simulink model "V2G_FDCC"  (R2024a)
settings: Solver=FixedStepAuto  StartTime=0.0  StopTime=10  FixedStep=1e-5  MaxStep=1.0E-5  RelTol=1e-3
values from neighbouring files (symbols this model uses):
  Batt_Ah = 2000    [main_v2gg2v.m]
  Batt_RespTime = 1    [main_v2gg2v.m]
  Batt_Vnom = 800    [main_v2gg2v.m]
  C_inv = (r*(Pinv/3)*al*(-be+al-1))/(100*Vac_l_rms*Vin_inv*wn*(al-be))    [main_v2gg2v.m]    (also in script.m = 0.00198943678865)
  C_mppt = 20*(Iout_mppt*D_mppt)/(deltaV*fs_mppt)    (= 0.0948148148148)    [main_v2gg2v.m]    (also in script.m)
  C_Vdc = 100*18e-3    (= 1.8)    [main_v2gg2v.m]
  cap_bat = 2000    [main_v2gg2v.m]    (also in script.m)
  Cbat_buck = deltaI_bat/(8*fs_bat*deltaV_bat)    (= 0.00133333333333)    [main_v2gg2v.m]    (also in script.m)
  Cdc = 30e-3    (= 0.03)    [main_v2gg2v.m]    (also in script.m)
  Cdc_boost = 50*Cbat_buck    (= 0.0666666666667)    [main_v2gg2v.m]    (also in script.m)
  Cf = 10*165e-6    (= 0.00165)    [main_v2gg2v.m]
  D = 2    [main_v2gg2v.m]
  Dinv = 0    [main_v2gg2v.m]
  f_grid = 50    [main_v2gg2v.m]
  fg = 50    [main_v2gg2v.m]    (also in script.m)
  H1 = 7    [main_v2gg2v.m]
  H2 = 8    [main_v2gg2v.m]
  H3 = 12    [main_v2gg2v.m]
  Hinv = 0    [main_v2gg2v.m]
  Ki_CC = 1    [main_v2gg2v.m]
  Ki_inner = 5000    [main_v2gg2v.m]
  Ki_outer = 10000    [main_v2gg2v.m]
  Ki_PLL = 10000    [main_v2gg2v.m]
  Kp_CC = 10    [main_v2gg2v.m]
  Kp_inner = 100    [main_v2gg2v.m]
  Kp_outer = 250    [main_v2gg2v.m]
  Kp_PLL = 100    [main_v2gg2v.m]
  L_bat = (Vbat*(Vdc_link-Vbat))/(deltaI_bat*fs_bat*Vdc_link)    (= 0.001875)    [main_v2gg2v.m]    (also in script.m)
  L_mppt = 1*(Vpv*D_mppt)/(deltaI*fs_mppt)    (= 0.000161333333333)    [main_v2gg2v.m]    (also in script.m)
  Lgrid = 1/10*0.69e-3    (= 6.9e-05)    [main_v2gg2v.m]
  Linv = 1/10*0.48e-3    (= 4.8e-05)    [main_v2gg2v.m]
  Lmin_inv = (100*Vac_l_rms*Vin_inv*(al-be))/(wn*r*(Pinv/3)*(-be+al-1))    [main_v2gg2v.m]    (also in script.m = 0.000611154981473)
  LowSat_CC = 0    [main_v2gg2v.m]
  omega = 2*pi*f_grid    (= 314.159265359)    [main_v2gg2v.m]
  Pinv = 2e6    (= 2000000)    [main_v2gg2v.m]    (also in script.m)
  Rd = 1.31    [main_v2gg2v.m]
  Sbase = 1e6    (= 1000000)    [main_v2gg2v.m]    (also in script.m)
  Snom_trafo = 1050e6    (= 1050000000)    [main_v2gg2v.m]
  t_fault_end = t_fault_start + FCT    (= 1.1)    [main_v2gg2v.m]
  t_fault_start = 1    [main_v2gg2v.m]
  Ts = 1e-5    (= 1e-05)    [main_v2gg2v.m]
  UpSat_CC = 1    [main_v2gg2v.m]
  Vac_inv = 800    [main_v2gg2v.m]    (also in script.m)
  Vbase = 345e3    (= 345000)    [main_v2gg2v.m]    (also in script.m)
  Vbat = 750    [main_v2gg2v.m]    (also in script.m)
  Vdc_ref = 1.5e3    (= 1500)    [main_v2gg2v.m]
  wg = 2*pi*fg    (= 314.159265359)    [main_v2gg2v.m]    (also in script.m)
undefined symbols (not defined in the file or in its folder): Acid, D1, Delta, h_PEV, Ibatfault_ref, ibatref, Ion, L12, L13, L23, Lbat, Lbuckboost, Lead, Lithium, R_Vdc, Rbuckboost, Vfault_thresh, vthref
libraries: spsSeriesRLCBranchLib x74, slpidlib x62, spsMosfetLib x50, spsGroundLib x48, spsBatteryLib x31, eeGeneralControl x31, spsPWMGeneratorDCDCLib x29, spsCurrentMeasurementLib x28, spsThreePhaseSeriesRLCBranchLib x21, spsThreePhaseVIMeasurementLib x18, spsIGBTDiodeLib x18, spsVoltageMeasurementLib x14
(part 9 of 11)

== system V2G_FDCC/V2G-G2V-1/5 Charging Stations/Charging Station5 ==
  Ibat_ref : Inport
  Battery : spsBatteryLib/Battery  BatType=Lithium-Ion  ShowTempParam=off  ThermalPreset=no  ShowAgeParam=off  NomV=Batt_Vnom  NomQ=Batt_Ah  SOC=Batt_InitSOC  Batt_Tr=Batt_RespTime  PresetModel=on  MaxQ=2000  MinV=600  FullV=931.1897  Dis_rate=869.5652  R=0.004  Normal_OP=1808.6957  expZone="[864.3087      98.26087]"  current=[6.5 13 32.5]  Units=Time  Tci=20  NomT=20  T2=-30  MaxQ2=4.8  FullV2=7.1  Normal_OP2=5.655  expZone2="[6.58           1]"  Rca=0.6  ti=2000  Dp=0  Neq0=0  Tsim=1e6  Ta1=25  Qeol=5.4*0.9  Reol=0.013333*1.2  Char_age=[2.3478, 3]  Dis_age=[2.3478, 10]  N1=1500  N2=10500  N3=1000  N4=1400  Ta2=45  N5=950
      settings: LibrarySourceBlock=electricdrivelib/Extra Sources/Battery
  Bus Selector : BusSelector  OutputSignals=SOC (%),Current (A),Voltage (V)
  Logical Operator : Logic  Operator=NOT  AllPortsSameDT=off  OutDataTypeStr=boolean
  Mosfet : spsMosfetLib/Mosfet  Ron=0.1  Lon=0  Rd=0.01  Vfd=0  IC=0  Rs=1e5  Cs=inf  Measurements=off
  Mosfet1 : spsMosfetLib/Mosfet  Ron=0.1  Lon=0  Rd=0.01  Vfd=0  IC=0  Rs=1e5  Cs=inf  Measurements=off
  PID Controller4 : slpidlib/PID Controller  Controller=PI  Form=Parallel  TimeDomain=Continuous-time  UseExternalTs=off  SampleTime=-1  IntegratorMethod=Forward Euler  FilterMethod=Forward Euler  ControllerParametersSource=internal  P=Kp_CC  I=Ki_CC  UseKiTs=off  D=0  UseExternalDerivativeSource=off  N=100  UseFilter=on  TunerSelectOption=Transfer Function Based (PID Tuner App)  ZeroCross=off  InitialConditionSource=internal  InitialConditionForIntegrator=0  InitialConditionForFilter=0  DifferentiatorICPrevScaledInput=0  ExternalReset=none  TrackingMode=off  Kt=1  LimitOutput=on  SatLimitsSource=internal  UpperSaturationLimit=UpSat_CC  LowerSaturationLimit=LowSat_CC  LinearizeAsGain=on  AntiWindupMode=none  Kb=1  LimitIntegrator=off  UpperIntegratorSaturationLimit=inf  LowerIntegratorSaturationLimit=-inf  POutMin=[]  POutMax=[]  IOutMin=[]  IOutMax=[]  DOutMin=[]  DOutMax=[]  NOutMin=[]  NOutMax=[]  SumOutMin=[]  SumOutMax=[]  SaturationOutMin=[]  SaturationOutMax=[]  PParamMin=[]  PParamMax=[]  IParamMin=[]  IParamMax=[]  DParamMin=[]  DParamMax=[]  NParamMin=[]  NParamMax=[]  KbParamMin=[]  KbParamMax=[]  KtParamMin=[]  KtParamMax=[]  KbOutMin=[]  KbOutMax=[]  KtOutMin=[]  KtOutMax=[]  IntegratorOutMin=[]  IntegratorOutMax=[]  FilterOutMin=[]  FilterOutMax=[]  SumI1OutMin=[]  SumI1OutMax=[]  SumI2OutMin=[]  SumI2OutMax=[]  SumI3OutMin=[]  SumI3OutMax=[]  SumI4OutMin=[]  SumI4OutMax=[]  SumDOutMin=[]  SumDOutMax=[]  DifferentiatorOutMin=[]  DifferentiatorOutMax=[]  FilterDiffOutCoefMin=[]  FilterDiffOutCoefMax=[]  ReciprocalOutMin=[]  ReciprocalOutMax=[]  SumDenOutMin=[]  SumDenOutMax=[]  SumNumOutMin=[]  SumNumOutMax=[]  DivideOutMin=[]  DivideOutMax=[]  UdiffTsProdOutMin=[]  UdiffTsProdOutMax=[]  NTsProdOutMin=[]  NTsProdOutMax=[]  UintegralTsProdOutMin=[]  UintegralTsProdOutMax=[]  UngainTsProdOutMin=[]  UngainTsProdOutMax=[]  ClampingZeroOutDataTypeStr=Inherit: Inherit via back propagation  ClampingZeroOutMin=[]  ClampingZeroOutMax=[]  FilterDenConstantOutDataTypeStr=Inherit: Inherit via back propagation  FilterDenConstantOutMin=[]  FilterDenConstantOutMax=[]  PCopyOutDataTypeStr=Inherit: Inherit via back propagation  PCopyOutMin=[]  PCopyOutMax=[]  NCopyOutDataTypeStr=Inherit: Inherit via back propagation  NCopyOutMin=[]  NCopyOutMax=[]  IntegratorContinuousStateAttributes=''  IntegratorStateMustResolveToSignalObject=off  IntegratorRTWStateStorageClass=Auto  FilterContinuousStateAttributes=''  FilterStateMustResolveToSignalObject=off  FilterRTWStateStorageClass=Auto  ParallelPVariant=InternalParameters  IdealPVariant=Disabled  IVariant=InternalParameters  DVariant=Disabled  IntegratorVariant=Continuous  SatVariant=Enabled  AWVariant=Passthrough  PCopyVariant=Disabled  TRVariant=Disabled  FdbkBlocksVariant=Forward  IdealPFdbkVariant=Disabled  SatFdbkVariant=Disabled  DerivativeFilterVariant=Disabled  NVariant=Disabled  NCopyVariant=Disabled_SignalSpec  FilterICVariant=Disabled  IntegratorICVariant=InternalICs  ExternalResetVariant=Disabled  TRSumVariant=Passthrough  SumFdbkVariant=Disabled  SumVariant=Sum_PI  TsampFilterVariant=InternalTs  TsampNgainVariant=Passthrough  TsampIntegralVariant=Disabled_SignalSpec  ExternalSaturationOutDataTypeStr=Inherit: Same as second input  DerivativeSourceVariant=Disabled
  PWM Generator (DC-DC) : spsPWMGeneratorDCDCLib/PWM Generator (DC-DC)  Fsw=f_SW  Ts=0
  Series RLC Branch9 : spsSeriesRLCBranchLib/Series RLC Branch  LConnTagsString=__new0  RConnTagsString=__new0  BranchType=L  Resistance=Rbuckboost  Inductance=Lbat  SetiL0=off  InitialCurrent=0  Capacitance=1e-6  Setx0=off  InitialVoltage=0  Measurements=None
  Sum8 : Sum  Inputs=|+-
  Terminator{,1..3} (4 alike) : Terminator
  VDC+ : PMIOPort  Side=Left
  VDC- : PMIOPort  Port=2  Side=Left
  wires:
  Bus Selector/3 -> Terminator3/1  "<Voltage (V)>"
  Bus Selector/2 -> Terminator2/1, [Ibat]  "<Current (A)>"
  [Buck] -> Mosfet/1
  Battery/1 -> Terminator/1, Bus Selector/1
  [Boost] -> Mosfet1/1
  Bus Selector/1 -> Terminator1/1  "<SOC (%)>"
  Logical Operator/1 -> [Boost]
  Ibat_ref/1 -> Sum8/2
  PID Controller4/1 -> PWM Generator (DC-DC)/1
  [Ibat] -> Sum8/1
  Sum8/1 -> PID Controller4/1
  PWM Generator (DC-DC)/1 -> Logical Operator/1, [Buck]
  connections:
  VDC-/RConn1 -- Battery/LConn2 -- Mosfet1/RConn1
  Mosfet/LConn1 -- VDC+/RConn1
  Mosfet1/LConn1 -- Series RLC Branch9/RConn1 -- Mosfet/RConn1
  Battery/LConn1 -- Series RLC Branch9/LConn1

== system V2G_FDCC/V2G-G2V-1/5 Charging Stations/Charging Station6 ==
  Ibat_ref : Inport
  Battery : spsBatteryLib/Battery  BatType=Lithium-Ion  ShowTempParam=off  ThermalPreset=no  ShowAgeParam=off  NomV=Batt_Vnom  NomQ=Batt_Ah  SOC=Batt_InitSOC  Batt_Tr=Batt_RespTime  PresetModel=on  MaxQ=2000  MinV=600  FullV=931.1897  Dis_rate=869.5652  R=0.004  Normal_OP=1808.6957  expZone="[864.3087      98.26087]"  current=[6.5 13 32.5]  Units=Time  Tci=20  NomT=20  T2=-30  MaxQ2=4.8  FullV2=7.1  Normal_OP2=5.655  expZone2="[6.58           1]"  Rca=0.6  ti=2000  Dp=0  Neq0=0  Tsim=1e6  Ta1=25  Qeol=5.4*0.9  Reol=0.013333*1.2  Char_age=[2.3478, 3]  Dis_age=[2.3478, 10]  N1=1500  N2=10500  N3=1000  N4=1400  Ta2=45  N5=950
      settings: LibrarySourceBlock=electricdrivelib/Extra Sources/Battery
  Bus Selector : BusSelector  OutputSignals=SOC (%),Current (A),Voltage (V)
  Logical Operator : Logic  Operator=NOT  AllPortsSameDT=off  OutDataTypeStr=boolean
  Mosfet : spsMosfetLib/Mosfet  Ron=0.1  Lon=0  Rd=0.01  Vfd=0  IC=0  Rs=1e5  Cs=inf  Measurements=off
  Mosfet1 : spsMosfetLib/Mosfet  Ron=0.1  Lon=0  Rd=0.01  Vfd=0  IC=0  Rs=1e5  Cs=inf  Measurements=off
  PID Controller4 : slpidlib/PID Controller  Controller=PI  Form=Parallel  TimeDomain=Continuous-time  UseExternalTs=off  SampleTime=-1  IntegratorMethod=Forward Euler  FilterMethod=Forward Euler  ControllerParametersSource=internal  P=Kp_CC  I=Ki_CC  UseKiTs=off  D=0  UseExternalDerivativeSource=off  N=100  UseFilter=on  TunerSelectOption=Transfer Function Based (PID Tuner App)  ZeroCross=off  InitialConditionSource=internal  InitialConditionForIntegrator=0  InitialConditionForFilter=0  DifferentiatorICPrevScaledInput=0  ExternalReset=none  TrackingMode=off  Kt=1  LimitOutput=on  SatLimitsSource=internal  UpperSaturationLimit=UpSat_CC  LowerSaturationLimit=LowSat_CC  LinearizeAsGain=on  AntiWindupMode=none  Kb=1  LimitIntegrator=off  UpperIntegratorSaturationLimit=inf  LowerIntegratorSaturationLimit=-inf  POutMin=[]  POutMax=[]  IOutMin=[]  IOutMax=[]  DOutMin=[]  DOutMax=[]  NOutMin=[]  NOutMax=[]  SumOutMin=[]  SumOutMax=[]  SaturationOutMin=[]  SaturationOutMax=[]  PParamMin=[]  PParamMax=[]  IParamMin=[]  IParamMax=[]  DParamMin=[]  DParamMax=[]  NParamMin=[]  NParamMax=[]  KbParamMin=[]  KbParamMax=[]  KtParamMin=[]  KtParamMax=[]  KbOutMin=[]  KbOutMax=[]  KtOutMin=[]  KtOutMax=[]  IntegratorOutMin=[]  IntegratorOutMax=[]  FilterOutMin=[]  FilterOutMax=[]  SumI1OutMin=[]  SumI1OutMax=[]  SumI2OutMin=[]  SumI2OutMax=[]  SumI3OutMin=[]  SumI3OutMax=[]  SumI4OutMin=[]  SumI4OutMax=[]  SumDOutMin=[]  SumDOutMax=[]  DifferentiatorOutMin=[]  DifferentiatorOutMax=[]  FilterDiffOutCoefMin=[]  FilterDiffOutCoefMax=[]  ReciprocalOutMin=[]  ReciprocalOutMax=[]  SumDenOutMin=[]  SumDenOutMax=[]  SumNumOutMin=[]  SumNumOutMax=[]  DivideOutMin=[]  DivideOutMax=[]  UdiffTsProdOutMin=[]  UdiffTsProdOutMax=[]  NTsProdOutMin=[]  NTsProdOutMax=[]  UintegralTsProdOutMin=[]  UintegralTsProdOutMax=[]  UngainTsProdOutMin=[]  UngainTsProdOutMax=[]  ClampingZeroOutDataTypeStr=Inherit: Inherit via back propagation  ClampingZeroOutMin=[]  ClampingZeroOutMax=[]  FilterDenConstantOutDataTypeStr=Inherit: Inherit via back propagation  FilterDenConstantOutMin=[]  FilterDenConstantOutMax=[]  PCopyOutDataTypeStr=Inherit: Inherit via back propagation  PCopyOutMin=[]  PCopyOutMax=[]  NCopyOutDataTypeStr=Inherit: Inherit via back propagation  NCopyOutMin=[]  NCopyOutMax=[]  IntegratorContinuousStateAttributes=''  IntegratorStateMustResolveToSignalObject=off  IntegratorRTWStateStorageClass=Auto  FilterContinuousStateAttributes=''  FilterStateMustResolveToSignalObject=off  FilterRTWStateStorageClass=Auto  ParallelPVariant=InternalParameters  IdealPVariant=Disabled  IVariant=InternalParameters  DVariant=Disabled  IntegratorVariant=Continuous  SatVariant=Enabled  AWVariant=Passthrough  PCopyVariant=Disabled  TRVariant=Disabled  FdbkBlocksVariant=Forward  IdealPFdbkVariant=Disabled  SatFdbkVariant=Disabled  DerivativeFilterVariant=Disabled  NVariant=Disabled  NCopyVariant=Disabled_SignalSpec  FilterICVariant=Disabled  IntegratorICVariant=InternalICs  ExternalResetVariant=Disabled  TRSumVariant=Passthrough  SumFdbkVariant=Disabled  SumVariant=Sum_PI  TsampFilterVariant=InternalTs  TsampNgainVariant=Passthrough  TsampIntegralVariant=Disabled_SignalSpec  ExternalSaturationOutDataTypeStr=Inherit: Same as second input  DerivativeSourceVariant=Disabled
  PWM Generator (DC-DC) : spsPWMGeneratorDCDCLib/PWM Generator (DC-DC)  Fsw=f_SW  Ts=0
  Series RLC Branch9 : spsSeriesRLCBranchLib/Series RLC Branch  LConnTagsString=__new0  RConnTagsString=__new0  BranchType=L  Resistance=Rbuckboost  Inductance=Lbat  SetiL0=off  InitialCurrent=0  Capacitance=1e-6  Setx0=off  InitialVoltage=0  Measurements=None
  Sum8 : Sum  Inputs=|+-
  Terminator{,1..3} (4 alike) : Terminator
  VDC+ : PMIOPort  Side=Left
  VDC- : PMIOPort  Port=2  Side=Left
  wires:
  Bus Selector/3 -> Terminator3/1  "<Voltage (V)>"
  Bus Selector/2 -> Terminator2/1, [Ibat]  "<Current (A)>"
  [Buck] -> Mosfet/1
  Battery/1 -> Terminator/1, Bus Selector/1
  [Boost] -> Mosfet1/1
  Bus Selector/1 -> Terminator1/1  "<SOC (%)>"
  Logical Operator/1 -> [Boost]
  Ibat_ref/1 -> Sum8/2
  PID Controller4/1 -> PWM Generator (DC-DC)/1
  [Ibat] -> Sum8/1
  Sum8/1 -> PID Controller4/1
  PWM Generator (DC-DC)/1 -> Logical Operator/1, [Buck]
  connections:
  VDC-/RConn1 -- Battery/LConn2 -- Mosfet1/RConn1
  Mosfet/LConn1 -- VDC+/RConn1
  Mosfet1/LConn1 -- Series RLC Branch9/RConn1 -- Mosfet/RConn1
  Battery/LConn1 -- Series RLC Branch9/LConn1

== system V2G_FDCC/V2G-G2V-1/5 Charging Stations/Charging Station7 ==
  Ibat_ref : Inport
  Battery : spsBatteryLib/Battery  BatType=Lithium-Ion  ShowTempParam=off  ThermalPreset=no  ShowAgeParam=off  NomV=Batt_Vnom  NomQ=Batt_Ah  SOC=Batt_InitSOC  Batt_Tr=Batt_RespTime  PresetModel=on  MaxQ=2000  MinV=600  FullV=931.1897  Dis_rate=869.5652  R=0.004  Normal_OP=1808.6957  expZone="[864.3087      98.26087]"  current=[6.5 13 32.5]  Units=Time  Tci=20  NomT=20  T2=-30  MaxQ2=4.8  FullV2=7.1  Normal_OP2=5.655  expZone2="[6.58           1]"  Rca=0.6  ti=2000  Dp=0  Neq0=0  Tsim=1e6  Ta1=25  Qeol=5.4*0.9  Reol=0.013333*1.2  Char_age=[2.3478, 3]  Dis_age=[2.3478, 10]  N1=1500  N2=10500  N3=1000  N4=1400  Ta2=45  N5=950
      settings: LibrarySourceBlock=electricdrivelib/Extra Sources/Battery
  Bus Selector : BusSelector  OutputSignals=SOC (%),Current (A),Voltage (V)
  Logical Operator : Logic  Operator=NOT  AllPortsSameDT=off  OutDataTypeStr=boolean
  Mosfet : spsMosfetLib/Mosfet  Ron=0.1  Lon=0  Rd=0.01  Vfd=0  IC=0  Rs=1e5  Cs=inf  Measurements=off
  Mosfet1 : spsMosfetLib/Mosfet  Ron=0.1  Lon=0  Rd=0.01  Vfd=0  IC=0  Rs=1e5  Cs=inf  Measurements=off
  PID Controller4 : slpidlib/PID Controller  Controller=PI  Form=Parallel  TimeDomain=Continuous-time  UseExternalTs=off  SampleTime=-1  IntegratorMethod=Forward Euler  FilterMethod=Forward Euler  ControllerParametersSource=internal  P=Kp_CC  I=Ki_CC  UseKiTs=off  D=0  UseExternalDerivativeSource=off  N=100  UseFilter=on  TunerSelectOption=Transfer Function Based (PID Tuner App)  ZeroCross=off  InitialConditionSource=internal  InitialConditionForIntegrator=0  InitialConditionForFilter=0  DifferentiatorICPrevScaledInput=0  ExternalReset=none  TrackingMode=off  Kt=1  LimitOutput=on  SatLimitsSource=internal  UpperSaturationLimit=UpSat_CC  LowerSaturationLimit=LowSat_CC  LinearizeAsGain=on  AntiWindupMode=none  Kb=1  LimitIntegrator=off  UpperIntegratorSaturationLimit=inf  LowerIntegratorSaturationLimit=-inf  POutMin=[]  POutMax=[]  IOutMin=[]  IOutMax=[]  DOutMin=[]  DOutMax=[]  NOutMin=[]  NOutMax=[]  SumOutMin=[]  SumOutMax=[]  SaturationOutMin=[]  SaturationOutMax=[]  PParamMin=[]  PParamMax=[]  IParamMin=[]  IParamMax=[]  DParamMin=[]  DParamMax=[]  NParamMin=[]  NParamMax=[]  KbParamMin=[]  KbParamMax=[]  KtParamMin=[]  KtParamMax=[]  KbOutMin=[]  KbOutMax=[]  KtOutMin=[]  KtOutMax=[]  IntegratorOutMin=[]  IntegratorOutMax=[]  FilterOutMin=[]  FilterOutMax=[]  SumI1OutMin=[]  SumI1OutMax=[]  SumI2OutMin=[]  SumI2OutMax=[]  SumI3OutMin=[]  SumI3OutMax=[]  SumI4OutMin=[]  SumI4OutMax=[]  SumDOutMin=[]  SumDOutMax=[]  DifferentiatorOutMin=[]  DifferentiatorOutMax=[]  FilterDiffOutCoefMin=[]  FilterDiffOutCoefMax=[]  ReciprocalOutMin=[]  ReciprocalOutMax=[]  SumDenOutMin=[]  SumDenOutMax=[]  SumNumOutMin=[]  SumNumOutMax=[]  DivideOutMin=[]  DivideOutMax=[]  UdiffTsProdOutMin=[]  UdiffTsProdOutMax=[]  NTsProdOutMin=[]  NTsProdOutMax=[]  UintegralTsProdOutMin=[]  UintegralTsProdOutMax=[]  UngainTsProdOutMin=[]  UngainTsProdOutMax=[]  ClampingZeroOutDataTypeStr=Inherit: Inherit via back propagation  ClampingZeroOutMin=[]  ClampingZeroOutMax=[]  FilterDenConstantOutDataTypeStr=Inherit: Inherit via back propagation  FilterDenConstantOutMin=[]  FilterDenConstantOutMax=[]  PCopyOutDataTypeStr=Inherit: Inherit via back propagation  PCopyOutMin=[]  PCopyOutMax=[]  NCopyOutDataTypeStr=Inherit: Inherit via back propagation  NCopyOutMin=[]  NCopyOutMax=[]  IntegratorContinuousStateAttributes=''  IntegratorStateMustResolveToSignalObject=off  IntegratorRTWStateStorageClass=Auto  FilterContinuousStateAttributes=''  FilterStateMustResolveToSignalObject=off  FilterRTWStateStorageClass=Auto  ParallelPVariant=InternalParameters  IdealPVariant=Disabled  IVariant=InternalParameters  DVariant=Disabled  IntegratorVariant=Continuous  SatVariant=Enabled  AWVariant=Passthrough  PCopyVariant=Disabled  TRVariant=Disabled  FdbkBlocksVariant=Forward  IdealPFdbkVariant=Disabled  SatFdbkVariant=Disabled  DerivativeFilterVariant=Disabled  NVariant=Disabled  NCopyVariant=Disabled_SignalSpec  FilterICVariant=Disabled  IntegratorICVariant=InternalICs  ExternalResetVariant=Disabled  TRSumVariant=Passthrough  SumFdbkVariant=Disabled  SumVariant=Sum_PI  TsampFilterVariant=InternalTs  TsampNgainVariant=Passthrough  TsampIntegralVariant=Disabled_SignalSpec  ExternalSaturationOutDataTypeStr=Inherit: Same as second input  DerivativeSourceVariant=Disabled
  PWM Generator (DC-DC) : spsPWMGeneratorDCDCLib/PWM Generator (DC-DC)  Fsw=f_SW  Ts=0
  Series RLC Branch9 : spsSeriesRLCBranchLib/Series RLC Branch  LConnTagsString=__new0  RConnTagsString=__new0  BranchType=L  Resistance=Rbuckboost  Inductance=Lbat  SetiL0=off  InitialCurrent=0  Capacitance=1e-6  Setx0=off  InitialVoltage=0  Measurements=None
  Sum8 : Sum  Inputs=|+-
  Terminator{,1..3} (4 alike) : Terminator
  VDC+ : PMIOPort  Side=Left
  VDC- : PMIOPort  Port=2  Side=Left
  wires:
  Bus Selector/3 -> Terminator3/1  "<Voltage (V)>"
  Bus Selector/2 -> Terminator2/1, [Ibat]  "<Current (A)>"
  [Buck] -> Mosfet/1
  Battery/1 -> Terminator/1, Bus Selector/1
  [Boost] -> Mosfet1/1
  Bus Selector/1 -> Terminator1/1  "<SOC (%)>"
  Logical Operator/1 -> [Boost]
  Ibat_ref/1 -> Sum8/2
  PID Controller4/1 -> PWM Generator (DC-DC)/1
  [Ibat] -> Sum8/1
  Sum8/1 -> PID Controller4/1
  PWM Generator (DC-DC)/1 -> Logical Operator/1, [Buck]
  connections:
  VDC-/RConn1 -- Battery/LConn2 -- Mosfet1/RConn1
  Mosfet/LConn1 -- VDC+/RConn1
  Mosfet1/LConn1 -- Series RLC Branch9/RConn1 -- Mosfet/RConn1
  Battery/LConn1 -- Series RLC Branch9/LConn1

== system V2G_FDCC/V2G-G2V-1/5 Charging Stations/Charging Station8 ==
  Ibat_ref : Inport
  Battery : spsBatteryLib/Battery  BatType=Lithium-Ion  ShowTempParam=off  ThermalPreset=no  ShowAgeParam=off  NomV=Batt_Vnom  NomQ=Batt_Ah  SOC=Batt_InitSOC  Batt_Tr=Batt_RespTime  PresetModel=on  MaxQ=2000  MinV=600  FullV=931.1897  Dis_rate=869.5652  R=0.004  Normal_OP=1808.6957  expZone="[864.3087      98.26087]"  current=[6.5 13 32.5]  Units=Time  Tci=20  NomT=20  T2=-30  MaxQ2=4.8  FullV2=7.1  Normal_OP2=5.655  expZone2="[6.58           1]"  Rca=0.6  ti=2000  Dp=0  Neq0=0  Tsim=1e6  Ta1=25  Qeol=5.4*0.9  Reol=0.013333*1.2  Char_age=[2.3478, 3]  Dis_age=[2.3478, 10]  N1=1500  N2=10500  N3=1000  N4=1400  Ta2=45  N5=950
      settings: LibrarySourceBlock=electricdrivelib/Extra Sources/Battery
  Bus Selector : BusSelector  OutputSignals=SOC (%),Current (A),Voltage (V)
  Logical Operator : Logic  Operator=NOT  AllPortsSameDT=off  OutDataTypeStr=boolean
  Mosfet : spsMosfetLib/Mosfet  Ron=0.1  Lon=0  Rd=0.01  Vfd=0  IC=0  Rs=1e5  Cs=inf  Measurements=off
  Mosfet1 : spsMosfetLib/Mosfet  Ron=0.1  Lon=0  Rd=0.01  Vfd=0  IC=0  Rs=1e5  Cs=inf  Measurements=off
  PID Controller4 : slpidlib/PID Controller  Controller=PI  Form=Parallel  TimeDomain=Continuous-time  UseExternalTs=off  SampleTime=-1  IntegratorMethod=Forward Euler  FilterMethod=Forward Euler  ControllerParametersSource=internal  P=Kp_CC  I=Ki_CC  UseKiTs=off  D=0  UseExternalDerivativeSource=off  N=100  UseFilter=on  TunerSelectOption=Transfer Function Based (PID Tuner App)  ZeroCross=off  InitialConditionSource=internal  InitialConditionForIntegrator=0  InitialConditionForFilter=0  DifferentiatorICPrevScaledInput=0  ExternalReset=none  TrackingMode=off  Kt=1  LimitOutput=on  SatLimitsSource=internal  UpperSaturationLimit=UpSat_CC  LowerSaturationLimit=LowSat_CC  LinearizeAsGain=on  AntiWindupMode=none  Kb=1  LimitIntegrator=off  UpperIntegratorSaturationLimit=inf  LowerIntegratorSaturationLimit=-inf  POutMin=[]  POutMax=[]  IOutMin=[]  IOutMax=[]  DOutMin=[]  DOutMax=[]  NOutMin=[]  NOutMax=[]  SumOutMin=[]  SumOutMax=[]  SaturationOutMin=[]  SaturationOutMax=[]  PParamMin=[]  PParamMax=[]  IParamMin=[]  IParamMax=[]  DParamMin=[]  DParamMax=[]  NParamMin=[]  NParamMax=[]  KbParamMin=[]  KbParamMax=[]  KtParamMin=[]  KtParamMax=[]  KbOutMin=[]  KbOutMax=[]  KtOutMin=[]  KtOutMax=[]  IntegratorOutMin=[]  IntegratorOutMax=[]  FilterOutMin=[]  FilterOutMax=[]  SumI1OutMin=[]  SumI1OutMax=[]  SumI2OutMin=[]  SumI2OutMax=[]  SumI3OutMin=[]  SumI3OutMax=[]  SumI4OutMin=[]  SumI4OutMax=[]  SumDOutMin=[]  SumDOutMax=[]  DifferentiatorOutMin=[]  DifferentiatorOutMax=[]  FilterDiffOutCoefMin=[]  FilterDiffOutCoefMax=[]  ReciprocalOutMin=[]  ReciprocalOutMax=[]  SumDenOutMin=[]  SumDenOutMax=[]  SumNumOutMin=[]  SumNumOutMax=[]  DivideOutMin=[]  DivideOutMax=[]  UdiffTsProdOutMin=[]  UdiffTsProdOutMax=[]  NTsProdOutMin=[]  NTsProdOutMax=[]  UintegralTsProdOutMin=[]  UintegralTsProdOutMax=[]  UngainTsProdOutMin=[]  UngainTsProdOutMax=[]  ClampingZeroOutDataTypeStr=Inherit: Inherit via back propagation  ClampingZeroOutMin=[]  ClampingZeroOutMax=[]  FilterDenConstantOutDataTypeStr=Inherit: Inherit via back propagation  FilterDenConstantOutMin=[]  FilterDenConstantOutMax=[]  PCopyOutDataTypeStr=Inherit: Inherit via back propagation  PCopyOutMin=[]  PCopyOutMax=[]  NCopyOutDataTypeStr=Inherit: Inherit via back propagation  NCopyOutMin=[]  NCopyOutMax=[]  IntegratorContinuousStateAttributes=''  IntegratorStateMustResolveToSignalObject=off  IntegratorRTWStateStorageClass=Auto  FilterContinuousStateAttributes=''  FilterStateMustResolveToSignalObject=off  FilterRTWStateStorageClass=Auto  ParallelPVariant=InternalParameters  IdealPVariant=Disabled  IVariant=InternalParameters  DVariant=Disabled  IntegratorVariant=Continuous  SatVariant=Enabled  AWVariant=Passthrough  PCopyVariant=Disabled  TRVariant=Disabled  FdbkBlocksVariant=Forward  IdealPFdbkVariant=Disabled  SatFdbkVariant=Disabled  DerivativeFilterVariant=Disabled  NVariant=Disabled  NCopyVariant=Disabled_SignalSpec  FilterICVariant=Disabled  IntegratorICVariant=InternalICs  ExternalResetVariant=Disabled  TRSumVariant=Passthrough  SumFdbkVariant=Disabled  SumVariant=Sum_PI  TsampFilterVariant=InternalTs  TsampNgainVariant=Passthrough  TsampIntegralVariant=Disabled_SignalSpec  ExternalSaturationOutDataTypeStr=Inherit: Same as second input  DerivativeSourceVariant=Disabled
  PWM Generator (DC-DC) : spsPWMGeneratorDCDCLib/PWM Generator (DC-DC)  Fsw=f_SW  Ts=0
  Series RLC Branch9 : spsSeriesRLCBranchLib/Series RLC Branch  LConnTagsString=__new0  RConnTagsString=__new0  BranchType=L  Resistance=Rbuckboost  Inductance=Lbat  SetiL0=off  InitialCurrent=0  Capacitance=1e-6  Setx0=off  InitialVoltage=0  Measurements=None
  Sum8 : Sum  Inputs=|+-
  Terminator{,1..3} (4 alike) : Terminator
  VDC+ : PMIOPort  Side=Left
  VDC- : PMIOPort  Port=2  Side=Left
  wires:
  Bus Selector/3 -> Terminator3/1  "<Voltage (V)>"
  Bus Selector/2 -> Terminator2/1, [Ibat]  "<Current (A)>"
  [Buck] -> Mosfet/1
  Battery/1 -> Terminator/1, Bus Selector/1
  [Boost] -> Mosfet1/1
  Bus Selector/1 -> Terminator1/1  "<SOC (%)>"
  Logical Operator/1 -> [Boost]
  Ibat_ref/1 -> Sum8/2
  PID Controller4/1 -> PWM Generator (DC-DC)/1
  [Ibat] -> Sum8/1
  Sum8/1 -> PID Controller4/1
  PWM Generator (DC-DC)/1 -> Logical Operator/1, [Buck]
  connections:
  VDC-/RConn1 -- Battery/LConn2 -- Mosfet1/RConn1
  Mosfet/LConn1 -- VDC+/RConn1
  Mosfet1/LConn1 -- Series RLC Branch9/RConn1 -- Mosfet/RConn1
  Battery/LConn1 -- Series RLC Branch9/LConn1

== system V2G_FDCC/V2G-G2V-1/5 Charging Stations/Charging Station9 ==
  Ibat_ref : Inport
  Battery : spsBatteryLib/Battery  BatType=Lithium-Ion  ShowTempParam=off  ThermalPreset=no  ShowAgeParam=off  NomV=Batt_Vnom  NomQ=Batt_Ah  SOC=Batt_InitSOC  Batt_Tr=Batt_RespTime  PresetModel=on  MaxQ=2000  MinV=600  FullV=931.1897  Dis_rate=869.5652  R=0.004  Normal_OP=1808.6957  expZone="[864.3087      98.26087]"  current=[6.5 13 32.5]  Units=Time  Tci=20  NomT=20  T2=-30  MaxQ2=4.8  FullV2=7.1  Normal_OP2=5.655  expZone2="[6.58           1]"  Rca=0.6  ti=2000  Dp=0  Neq0=0  Tsim=1e6  Ta1=25  Qeol=5.4*0.9  Reol=0.013333*1.2  Char_age=[2.3478, 3]  Dis_age=[2.3478, 10]  N1=1500  N2=10500  N3=1000  N4=1400  Ta2=45  N5=950
      settings: LibrarySourceBlock=electricdrivelib/Extra Sources/Battery
  Bus Selector : BusSelector  OutputSignals=SOC (%),Current (A),Voltage (V)
  Logical Operator : Logic  Operator=NOT  AllPortsSameDT=off  OutDataTypeStr=boolean
  Mosfet : spsMosfetLib/Mosfet  Ron=0.1  Lon=0  Rd=0.01  Vfd=0  IC=0  Rs=1e5  Cs=inf  Measurements=off
  Mosfet1 : spsMosfetLib/Mosfet  Ron=0.1  Lon=0  Rd=0.01  Vfd=0  IC=0  Rs=1e5  Cs=inf  Measurements=off
  PID Controller4 : slpidlib/PID Controller  Controller=PI  Form=Parallel  TimeDomain=Continuous-time  UseExternalTs=off  SampleTime=-1  IntegratorMethod=Forward Euler  FilterMethod=Forward Euler  ControllerParametersSource=internal  P=Kp_CC  I=Ki_CC  UseKiTs=off  D=0  UseExternalDerivativeSource=off  N=100  UseFilter=on  TunerSelectOption=Transfer Function Based (PID Tuner App)  ZeroCross=off  InitialConditionSource=internal  InitialConditionForIntegrator=0  InitialConditionForFilter=0  DifferentiatorICPrevScaledInput=0  ExternalReset=none  TrackingMode=off  Kt=1  LimitOutput=on  SatLimitsSource=internal  UpperSaturationLimit=UpSat_CC  LowerSaturationLimit=LowSat_CC  LinearizeAsGain=on  AntiWindupMode=none  Kb=1  LimitIntegrator=off  UpperIntegratorSaturationLimit=inf  LowerIntegratorSaturationLimit=-inf  POutMin=[]  POutMax=[]  IOutMin=[]  IOutMax=[]  DOutMin=[]  DOutMax=[]  NOutMin=[]  NOutMax=[]  SumOutMin=[]  SumOutMax=[]  SaturationOutMin=[]  SaturationOutMax=[]  PParamMin=[]  PParamMax=[]  IParamMin=[]  IParamMax=[]  DParamMin=[]  DParamMax=[]  NParamMin=[]  NParamMax=[]  KbParamMin=[]  KbParamMax=[]  KtParamMin=[]  KtParamMax=[]  KbOutMin=[]  KbOutMax=[]  KtOutMin=[]  KtOutMax=[]  IntegratorOutMin=[]  IntegratorOutMax=[]  FilterOutMin=[]  FilterOutMax=[]  SumI1OutMin=[]  SumI1OutMax=[]  SumI2OutMin=[]  SumI2OutMax=[]  SumI3OutMin=[]  SumI3OutMax=[]  SumI4OutMin=[]  SumI4OutMax=[]  SumDOutMin=[]  SumDOutMax=[]  DifferentiatorOutMin=[]  DifferentiatorOutMax=[]  FilterDiffOutCoefMin=[]  FilterDiffOutCoefMax=[]  ReciprocalOutMin=[]  ReciprocalOutMax=[]  SumDenOutMin=[]  SumDenOutMax=[]  SumNumOutMin=[]  SumNumOutMax=[]  DivideOutMin=[]  DivideOutMax=[]  UdiffTsProdOutMin=[]  UdiffTsProdOutMax=[]  NTsProdOutMin=[]  NTsProdOutMax=[]  UintegralTsProdOutMin=[]  UintegralTsProdOutMax=[]  UngainTsProdOutMin=[]  UngainTsProdOutMax=[]  ClampingZeroOutDataTypeStr=Inherit: Inherit via back propagation  ClampingZeroOutMin=[]  ClampingZeroOutMax=[]  FilterDenConstantOutDataTypeStr=Inherit: Inherit via back propagation  FilterDenConstantOutMin=[]  FilterDenConstantOutMax=[]  PCopyOutDataTypeStr=Inherit: Inherit via back propagation  PCopyOutMin=[]  PCopyOutMax=[]  NCopyOutDataTypeStr=Inherit: Inherit via back propagation  NCopyOutMin=[]  NCopyOutMax=[]  IntegratorContinuousStateAttributes=''  IntegratorStateMustResolveToSignalObject=off  IntegratorRTWStateStorageClass=Auto  FilterContinuousStateAttributes=''  FilterStateMustResolveToSignalObject=off  FilterRTWStateStorageClass=Auto  ParallelPVariant=InternalParameters  IdealPVariant=Disabled  IVariant=InternalParameters  DVariant=Disabled  IntegratorVariant=Continuous  SatVariant=Enabled  AWVariant=Passthrough  PCopyVariant=Disabled  TRVariant=Disabled  FdbkBlocksVariant=Forward  IdealPFdbkVariant=Disabled  SatFdbkVariant=Disabled  DerivativeFilterVariant=Disabled  NVariant=Disabled  NCopyVariant=Disabled_SignalSpec  FilterICVariant=Disabled  IntegratorICVariant=InternalICs  ExternalResetVariant=Disabled  TRSumVariant=Passthrough  SumFdbkVariant=Disabled  SumVariant=Sum_PI  TsampFilterVariant=InternalTs  TsampNgainVariant=Passthrough  TsampIntegralVariant=Disabled_SignalSpec  ExternalSaturationOutDataTypeStr=Inherit: Same as second input  DerivativeSourceVariant=Disabled
  PWM Generator (DC-DC) : spsPWMGeneratorDCDCLib/PWM Generator (DC-DC)  Fsw=f_SW  Ts=0
  Series RLC Branch9 : spsSeriesRLCBranchLib/Series RLC Branch  LConnTagsString=__new0  RConnTagsString=__new0  BranchType=L  Resistance=Rbuckboost  Inductance=Lbat  SetiL0=off  InitialCurrent=0  Capacitance=1e-6  Setx0=off  InitialVoltage=0  Measurements=None
  Sum8 : Sum  Inputs=|+-
  Terminator{,1..3} (4 alike) : Terminator
  VDC+ : PMIOPort  Side=Left
  VDC- : PMIOPort  Port=2  Side=Left
  wires:
  Bus Selector/3 -> Terminator3/1  "<Voltage (V)>"
  Bus Selector/2 -> Terminator2/1, [Ibat]  "<Current (A)>"
  [Buck] -> Mosfet/1
  Battery/1 -> Terminator/1, Bus Selector/1
  [Boost] -> Mosfet1/1
  Bus Selector/1 -> Terminator1/1  "<SOC (%)>"
  Logical Operator/1 -> [Boost]
  Ibat_ref/1 -> Sum8/2
  PID Controller4/1 -> PWM Generator (DC-DC)/1
  [Ibat] -> Sum8/1
  Sum8/1 -> PID Controller4/1
  PWM Generator (DC-DC)/1 -> Logical Operator/1, [Buck]
  connections:
  VDC-/RConn1 -- Battery/LConn2 -- Mosfet1/RConn1
  Mosfet/LConn1 -- VDC+/RConn1
  Mosfet1/LConn1 -- Series RLC Branch9/RConn1 -- Mosfet/RConn1
  Battery/LConn1 -- Series RLC Branch9/LConn1

== system V2G_FDCC/V2G-G2V-1/AC//DC Converter/Subsystem ==
  PWM1 : Inport
  PWM2 : Inport  Port=2
  PWM3 : Inport  Port=3
  PWM4 : Inport  Port=4
  PWM5 : Inport  Port=5
  PWM6 : Inport  Port=6
  IGBT/Diode{,1..5} (6 alike) : spsIGBTDiodeLib/IGBT//Diode  Ron=1e-3  Rs=1e5  Cs=inf  Measurements=off
  VR : PMIOPort  Side=Left
  VY : PMIOPort  Port=2  Side=Left
  VB : PMIOPort  Port=3  Side=Left
  VDC+ : PMIOPort  Port=4  Side=Right
  VDC- : PMIOPort  Port=5  Side=Right
  wires:
  PWM1/1 -> IGBT/Diode/1
  PWM5/1 -> IGBT/Diode4/1
  PWM4/1 -> IGBT/Diode3/1
  PWM6/1 -> IGBT/Diode5/1
  PWM3/1 -> IGBT/Diode2/1
  PWM2/1 -> IGBT/Diode1/1
  connections:
  IGBT/Diode4/RConn1 -- VB/RConn1 -- IGBT/Diode5/LConn1
  IGBT/Diode1/RConn1 -- IGBT/Diode3/RConn1 -- VDC-/RConn1 -- IGBT/Diode5/RConn1
  IGBT/Diode/RConn1 -- VR/RConn1 -- IGBT/Diode1/LConn1
  IGBT/Diode2/RConn1 -- VY/RConn1 -- IGBT/Diode3/LConn1
  IGBT/Diode/LConn1 -- VDC+/RConn1 -- IGBT/Diode4/LConn1 -- IGBT/Diode2/LConn1

== system V2G_FDCC/V2G-G2V-3/AC//DC Converter/Subsystem ==
  PWM1 : Inport
  PWM2 : Inport  Port=2
  PWM3 : Inport  Port=3
  PWM4 : Inport  Port=4
  PWM5 : Inport  Port=5
  PWM6 : Inport  Port=6
  IGBT/Diode{,1..5} (6 alike) : spsIGBTDiodeLib/IGBT//Diode  Ron=1e-3  Rs=1e5  Cs=inf  Measurements=off
  VR : PMIOPort  Side=Left
  VY : PMIOPort  Port=2  Side=Left
  VB : PMIOPort  Port=3  Side=Left
  VDC+ : PMIOPort  Port=4  Side=Right
  VDC- : PMIOPort  Port=5  Side=Right
  wires:
  PWM1/1 -> IGBT/Diode/1
  PWM5/1 -> IGBT/Diode4/1
  PWM4/1 -> IGBT/Diode3/1
  PWM6/1 -> IGBT/Diode5/1
  PWM3/1 -> IGBT/Diode2/1
  PWM2/1 -> IGBT/Diode1/1
  connections:
  IGBT/Diode4/RConn1 -- VB/RConn1 -- IGBT/Diode5/LConn1
  IGBT/Diode1/RConn1 -- IGBT/Diode3/RConn1 -- VDC-/RConn1 -- IGBT/Diode5/RConn1
  IGBT/Diode/RConn1 -- VR/RConn1 -- IGBT/Diode1/LConn1
  IGBT/Diode2/RConn1 -- VY/RConn1 -- IGBT/Diode3/LConn1
  IGBT/Diode/LConn1 -- VDC+/RConn1 -- IGBT/Diode4/LConn1 -- IGBT/Diode2/LConn1

== system V2G_FDCC/V2G-G2V-3/Charging Stations/Charging Station ==
  Ibat_ref : Inport
  5 EVs : spsBatteryLib/Battery  BatType=Lithium-Ion  ShowTempParam=off  ThermalPreset=no  ShowAgeParam=off  NomV=Batt_Vnom  NomQ=Batt_Ah*10  SOC=Batt_InitSOC  Batt_Tr=Batt_RespTime  PresetModel=on  MaxQ=20000  MinV=600  FullV=931.1897  Dis_rate=8695.6522  R=0.0004  Normal_OP=18086.9565  expZone="[864.3087      982.6087]"  current=[6.5 13 32.5]  Units=Time  Tci=20  NomT=20  T2=-30  MaxQ2=4.8  FullV2=7.1  Normal_OP2=5.655  expZone2="[6.58           1]"  Rca=0.6  ti=2000  Dp=0  Neq0=0  Tsim=1e6  Ta1=25  Qeol=5.4*0.9  Reol=0.013333*1.2  Char_age=[2.3478, 3]  Dis_age=[2.3478, 10]  N1=1500  N2=10500  N3=1000  N4=1400  Ta2=45  N5=950
      settings: LibrarySourceBlock=electricdrivelib/Extra Sources/Battery
  Bus Selector : BusSelector  OutputSignals=SOC (%),Current (A),Voltage (V)
  Logical Operator : Logic  Operator=NOT  AllPortsSameDT=off  OutDataTypeStr=boolean
  Mosfet : spsMosfetLib/Mosfet  Ron=0.1  Lon=0  Rd=0.01  Vfd=0  IC=0  Rs=1e5  Cs=inf  Measurements=off
  Mosfet1 : spsMosfetLib/Mosfet  Ron=0.1  Lon=0  Rd=0.01  Vfd=0  IC=0  Rs=1e5  Cs=inf  Measurements=off
  PID Controller4 : slpidlib/PID Controller  Controller=PI  Form=Parallel  TimeDomain=Continuous-time  UseExternalTs=off  SampleTime=-1  IntegratorMethod=Forward Euler  FilterMethod=Forward Euler  ControllerParametersSource=internal  P=Kp_CC  I=Ki_CC  UseKiTs=off  D=0  UseExternalDerivativeSource=off  N=100  UseFilter=on  TunerSelectOption=Transfer Function Based (PID Tuner App)  ZeroCross=off  InitialConditionSource=internal  InitialConditionForIntegrator=0  InitialConditionForFilter=0  DifferentiatorICPrevScaledInput=0  ExternalReset=none  TrackingMode=off  Kt=1  LimitOutput=on  SatLimitsSource=internal  UpperSaturationLimit=UpSat_CC  LowerSaturationLimit=LowSat_CC  LinearizeAsGain=on  AntiWindupMode=none  Kb=1  LimitIntegrator=off  UpperIntegratorSaturationLimit=inf  LowerIntegratorSaturationLimit=-inf  POutMin=[]  POutMax=[]  IOutMin=[]  IOutMax=[]  DOutMin=[]  DOutMax=[]  NOutMin=[]  NOutMax=[]  SumOutMin=[]  SumOutMax=[]  SaturationOutMin=[]  SaturationOutMax=[]  PParamMin=[]  PParamMax=[]  IParamMin=[]  IParamMax=[]  DParamMin=[]  DParamMax=[]  NParamMin=[]  NParamMax=[]  KbParamMin=[]  KbParamMax=[]  KtParamMin=[]  KtParamMax=[]  KbOutMin=[]  KbOutMax=[]  KtOutMin=[]  KtOutMax=[]  IntegratorOutMin=[]  IntegratorOutMax=[]  FilterOutMin=[]  FilterOutMax=[]  SumI1OutMin=[]  SumI1OutMax=[]  SumI2OutMin=[]  SumI2OutMax=[]  SumI3OutMin=[]  SumI3OutMax=[]  SumI4OutMin=[]  SumI4OutMax=[]  SumDOutMin=[]  SumDOutMax=[]  DifferentiatorOutMin=[]  DifferentiatorOutMax=[]  FilterDiffOutCoefMin=[]  FilterDiffOutCoefMax=[]  ReciprocalOutMin=[]  ReciprocalOutMax=[]  SumDenOutMin=[]  SumDenOutMax=[]  SumNumOutMin=[]  SumNumOutMax=[]  DivideOutMin=[]  DivideOutMax=[]  UdiffTsProdOutMin=[]  UdiffTsProdOutMax=[]  NTsProdOutMin=[]  NTsProdOutMax=[]  UintegralTsProdOutMin=[]  UintegralTsProdOutMax=[]  UngainTsProdOutMin=[]  UngainTsProdOutMax=[]  ClampingZeroOutDataTypeStr=Inherit: Inherit via back propagation  ClampingZeroOutMin=[]  ClampingZeroOutMax=[]  FilterDenConstantOutDataTypeStr=Inherit: Inherit via back propagation  FilterDenConstantOutMin=[]  FilterDenConstantOutMax=[]  PCopyOutDataTypeStr=Inherit: Inherit via back propagation  PCopyOutMin=[]  PCopyOutMax=[]  NCopyOutDataTypeStr=Inherit: Inherit via back propagation  NCopyOutMin=[]  NCopyOutMax=[]  IntegratorContinuousStateAttributes=''  IntegratorStateMustResolveToSignalObject=off  IntegratorRTWStateStorageClass=Auto  FilterContinuousStateAttributes=''  FilterStateMustResolveToSignalObject=off  FilterRTWStateStorageClass=Auto  ParallelPVariant=InternalParameters  IdealPVariant=Disabled  IVariant=InternalParameters  DVariant=Disabled  IntegratorVariant=Continuous  SatVariant=Enabled  AWVariant=Passthrough  PCopyVariant=Disabled  TRVariant=Disabled  FdbkBlocksVariant=Forward  IdealPFdbkVariant=Disabled  SatFdbkVariant=Disabled  DerivativeFilterVariant=Disabled  NVariant=Disabled  NCopyVariant=Disabled_SignalSpec  FilterICVariant=Disabled  IntegratorICVariant=InternalICs  ExternalResetVariant=Disabled  TRSumVariant=Passthrough  SumFdbkVariant=Disabled  SumVariant=Sum_PI  TsampFilterVariant=InternalTs  TsampNgainVariant=Passthrough  TsampIntegralVariant=Disabled_SignalSpec  ExternalSaturationOutDataTypeStr=Inherit: Same as second input  DerivativeSourceVariant=Disabled
  PWM Generator (DC-DC) : spsPWMGeneratorDCDCLib/PWM Generator (DC-DC)  Fsw=f_SW  Ts=0
  Series RLC Branch9 : spsSeriesRLCBranchLib/Series RLC Branch  LConnTagsString=__new0  RConnTagsString=__new0  BranchType=L  Resistance=Rbuckboost  Inductance=Lbat  SetiL0=off  InitialCurrent=0  Capacitance=1e-6  Setx0=off  InitialVoltage=0  Measurements=None
  Sum8 : Sum  Inputs=|+-
  VDC+ : PMIOPort  Side=Left
  VDC- : PMIOPort  Port=2  Side=Left
  to_workspace : Outport
  SOC : Outport  Port=2
  Current : Outport  Port=3
  Voltage : Outport  Port=4
  wires:
  Bus Selector/3 -> Voltage/1  "<Voltage (V)>"
  Bus Selector/2 -> [Ibat], Current/1  "<Current (A)>"
  [Buck] -> Mosfet/1
  5 EVs/1 -> to_workspace/1, Bus Selector/1
  [Boost] -> Mosfet1/1
  Bus Selector/1 -> SOC/1  "<SOC (%)>"
  Logical Operator/1 -> [Boost]
  Ibat_ref/1 -> Sum8/2
  PID Controller4/1 -> PWM Generator (DC-DC)/1
  [Ibat] -> Sum8/1
  Sum8/1 -> PID Controller4/1
  PWM Generator (DC-DC)/1 -> Logical Operator/1, [Buck]
  connections:
  VDC-/RConn1 -- 5 EVs/LConn2 -- Mosfet1/RConn1
  Mosfet/LConn1 -- VDC+/RConn1
  Mosfet1/LConn1 -- Series RLC Branch9/RConn1 -- Mosfet/RConn1
  5 EVs/LConn1 -- Series RLC Branch9/LConn1

== system V2G_FDCC/V2G-G2V-6/5 Charging Stations/Charging Station1 ==
  Ibat_ref : Inport
  Battery : spsBatteryLib/Battery  BatType=Lithium-Ion  ShowTempParam=off  ThermalPreset=no  ShowAgeParam=off  NomV=Batt_Vnom  NomQ=Batt_Ah  SOC=Batt_InitSOC  Batt_Tr=Batt_RespTime*0  PresetModel=on  MaxQ=2000  MinV=600  FullV=931.1897  Dis_rate=869.5652  R=0.004  Normal_OP=1808.6957  expZone="[864.3087      98.26087]"  current=[6.5 13 32.5]  Units=Time  Tci=20  NomT=20  T2=-30  MaxQ2=4.8  FullV2=7.1  Normal_OP2=5.655  expZone2="[6.58           1]"  Rca=0.6  ti=2000  Dp=0  Neq0=0  Tsim=1e6  Ta1=25  Qeol=5.4*0.9  Reol=0.013333*1.2  Char_age=[2.3478, 3]  Dis_age=[2.3478, 10]  N1=1500  N2=10500  N3=1000  N4=1400  Ta2=45  N5=950
      settings: LibrarySourceBlock=electricdrivelib/Extra Sources/Battery
  Bus Selector : BusSelector  OutputSignals=SOC (%),Current (A),Voltage (V)
  Current Measurement : spsCurrentMeasurementLib/Current Measurement  PhasorSimulation=off  OutputType=Complex  PSBequivalent=0
  Logical Operator : Logic  Operator=NOT  AllPortsSameDT=off  OutDataTypeStr=boolean
  Mosfet : spsMosfetLib/Mosfet  Ron=0.1  Lon=0  Rd=0.01  Vfd=0  IC=0  Rs=1e5  Cs=inf  Measurements=off
  Mosfet1 : spsMosfetLib/Mosfet  Ron=0.1  Lon=0  Rd=0.01  Vfd=0  IC=0  Rs=1e5  Cs=inf  Measurements=off
  PID Controller4 : slpidlib/PID Controller  Controller=PI  Form=Parallel  TimeDomain=Continuous-time  UseExternalTs=off  SampleTime=-1  IntegratorMethod=Forward Euler  FilterMethod=Forward Euler  ControllerParametersSource=internal  P=Kp_CC  I=Ki_CC  UseKiTs=off  D=0  UseExternalDerivativeSource=off  N=100  UseFilter=on  TunerSelectOption=Transfer Function Based (PID Tuner App)  ZeroCross=off  InitialConditionSource=internal  InitialConditionForIntegrator=0  InitialConditionForFilter=0  DifferentiatorICPrevScaledInput=0  ExternalReset=none  TrackingMode=off  Kt=1  LimitOutput=on  SatLimitsSource=internal  UpperSaturationLimit=UpSat_CC  LowerSaturationLimit=LowSat_CC  LinearizeAsGain=on  AntiWindupMode=none  Kb=1  LimitIntegrator=off  UpperIntegratorSaturationLimit=inf  LowerIntegratorSaturationLimit=-inf  POutMin=[]  POutMax=[]  IOutMin=[]  IOutMax=[]  DOutMin=[]  DOutMax=[]  NOutMin=[]  NOutMax=[]  SumOutMin=[]  SumOutMax=[]  SaturationOutMin=[]  SaturationOutMax=[]  PParamMin=[]  PParamMax=[]  IParamMin=[]  IParamMax=[]  DParamMin=[]  DParamMax=[]  NParamMin=[]  NParamMax=[]  KbParamMin=[]  KbParamMax=[]  KtParamMin=[]  KtParamMax=[]  KbOutMin=[]  KbOutMax=[]  KtOutMin=[]  KtOutMax=[]  IntegratorOutMin=[]  IntegratorOutMax=[]  FilterOutMin=[]  FilterOutMax=[]  SumI1OutMin=[]  SumI1OutMax=[]  SumI2OutMin=[]  SumI2OutMax=[]  SumI3OutMin=[]  SumI3OutMax=[]  SumI4OutMin=[]  SumI4OutMax=[]  SumDOutMin=[]  SumDOutMax=[]  DifferentiatorOutMin=[]  DifferentiatorOutMax=[]  FilterDiffOutCoefMin=[]  FilterDiffOutCoefMax=[]  ReciprocalOutMin=[]  ReciprocalOutMax=[]  SumDenOutMin=[]  SumDenOutMax=[]  SumNumOutMin=[]  SumNumOutMax=[]  DivideOutMin=[]  DivideOutMax=[]  UdiffTsProdOutMin=[]  UdiffTsProdOutMax=[]  NTsProdOutMin=[]  NTsProdOutMax=[]  UintegralTsProdOutMin=[]  UintegralTsProdOutMax=[]  UngainTsProdOutMin=[]  UngainTsProdOutMax=[]  ClampingZeroOutDataTypeStr=Inherit: Inherit via back propagation  ClampingZeroOutMin=[]  ClampingZeroOutMax=[]  FilterDenConstantOutDataTypeStr=Inherit: Inherit via back propagation  FilterDenConstantOutMin=[]  FilterDenConstantOutMax=[]  PCopyOutDataTypeStr=Inherit: Inherit via back propagation  PCopyOutMin=[]  PCopyOutMax=[]  NCopyOutDataTypeStr=Inherit: Inherit via back propagation  NCopyOutMin=[]  NCopyOutMax=[]  IntegratorContinuousStateAttributes=''  IntegratorStateMustResolveToSignalObject=off  IntegratorRTWStateStorageClass=Auto  FilterContinuousStateAttributes=''  FilterStateMustResolveToSignalObject=off  FilterRTWStateStorageClass=Auto  ParallelPVariant=InternalParameters  IdealPVariant=Disabled  IVariant=InternalParameters  DVariant=Disabled  IntegratorVariant=Continuous  SatVariant=Enabled  AWVariant=Passthrough  PCopyVariant=Disabled  TRVariant=Disabled  FdbkBlocksVariant=Forward  IdealPFdbkVariant=Disabled  SatFdbkVariant=Disabled  DerivativeFilterVariant=Disabled  NVariant=Disabled  NCopyVariant=Disabled_SignalSpec  FilterICVariant=Disabled  IntegratorICVariant=InternalICs  ExternalResetVariant=Disabled  TRSumVariant=Passthrough  SumFdbkVariant=Disabled  SumVariant=Sum_PI  TsampFilterVariant=InternalTs  TsampNgainVariant=Passthrough  TsampIntegralVariant=Disabled_SignalSpec  ExternalSaturationOutDataTypeStr=Inherit: Same as second input  DerivativeSourceVariant=Disabled
  PWM Generator (DC-DC) : spsPWMGeneratorDCDCLib/PWM Generator (DC-DC)  Fsw=f_SW  Ts=0
  Series RLC Branch9 : spsSeriesRLCBranchLib/Series RLC Branch  LConnTagsString=__new0  RConnTagsString=__new0  BranchType=L  Resistance=Rbuckboost  Inductance=L_bat  SetiL0=off  InitialCurrent=0  Capacitance=1e-6  Setx0=off  InitialVoltage=0  Measurements=None
  Sum8 : Sum  Inputs=|+-
  VDC+ : PMIOPort  Side=Left
  VDC- : PMIOPort  Port=2  Side=Left
  to_workspace : Outport
  SOC : Outport  Port=2
  Current : Outport  Port=3
  Voltage : Outport  Port=4
  wires:
  Bus Selector/3 -> Voltage/1  "<Voltage (V)>"
  Bus Selector/2 -> ?  "<Current (A)>"
  [Buck] -> Mosfet/1
  Battery/1 -> to_workspace/1, Bus Selector/1
  [Boost] -> Mosfet1/1
  Bus Selector/1 -> SOC/1  "<SOC (%)>"
  Logical Operator/1 -> [Boost]
  Ibat_ref/1 -> Sum8/2
  PID Controller4/1 -> PWM Generator (DC-DC)/1
  [Ibat] -> Sum8/1
  Sum8/1 -> PID Controller4/1
  PWM Generator (DC-DC)/1 -> Logical Operator/1, [Buck]
  Current Measurement/1 -> Current/1, [Ibat]
  connections:
  VDC-/RConn1 -- Battery/LConn2 -- Mosfet1/RConn1
  Mosfet/LConn1 -- VDC+/RConn1
  Mosfet1/LConn1 -- Series RLC Branch9/RConn1 -- Mosfet/RConn1
  Current Measurement/RConn1 -- Series RLC Branch9/LConn1
  Current Measurement/LConn1 -- Battery/LConn1
